simulink model "CoVM_TrqAcsCoord"  (R2016b)
settings: configuration reference "CodeGenConfigSet" (kept outside this file)
values from neighbouring files (symbols this model uses):
  TRQ_ZERO = uint16(0)    [init_CoVM_TrqAcsCoord.m]
settings Model: Creator=Administrator  LastModifiedBy=Wei Liang
settings ConfigSetRef: SourceLocation=Base Workspace

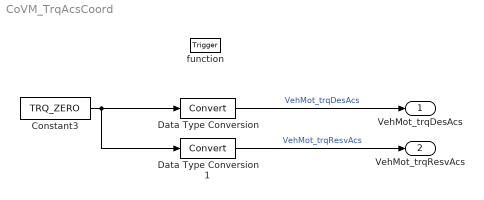
== system CoVM_TrqAcsCoord ==
  function : TriggerPort  TriggerType=function-call  VariantControl=Variant
  Constant3 : Constant  Description=Zero Torque  Value=TRQ_ZERO  OutDataTypeStr=Trq_Nm
  Data Type Conversion : DataTypeConversion
  Data Type Conversion1 : DataTypeConversion
  VehMot_trqDesAcs : Outport  Tag=Nm  Description=Required engine speed of Vehicle Motion acsessories  OutMin=-3000  OutMax=3000  OutDataTypeStr=Trq_Nm
  VehMot_trqResvAcs : Outport  Tag=Nm  Description=Demanded engine speed reserve by acsessories of Vehicle Motion  Port=2  OutMin=-3000  OutMax=3000  OutDataTypeStr=Trq_Nm
  wires:
  Constant3/1 -> Data Type Conversion1/1, Data Type Conversion/1
  Data Type Conversion/1 -> VehMot_trqDesAcs/1  "VehMot_trqDesAcs"
  Data Type Conversion1/1 -> VehMot_trqResvAcs/1  "VehMot_trqResvAcs"
